simulink model "inverse_shapers"  (R2015b)
settings: Solver=ode1  StartTime=0.0  StopTime=30  FixedStep=0.001  RelTol=1e-3
undefined symbols (not defined in the file): a, A, tau, tau_add, tau_sub
libraries: cstblocks x1
settings Model: Creator=dave  LastModifiedBy=dave

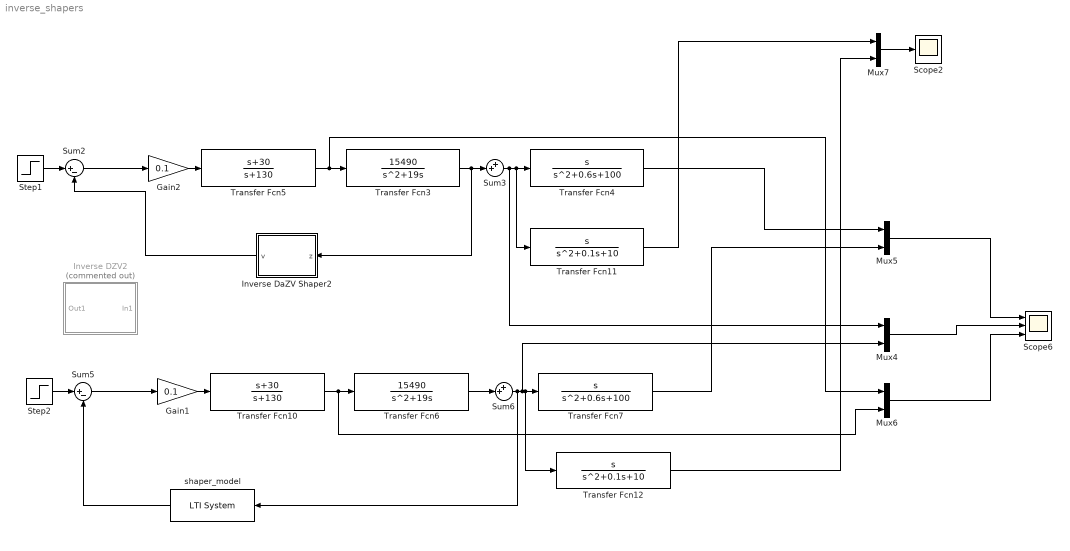
== system inverse_shapers ==
  Gain1 : Gain  Gain=0.1
  Gain2 : Gain  Gain=0.1
  Inverse DZV2 : Subsystem  Commented=on
  Inverse DaZV Shaper2 : Subsystem
  Mux{4..7} (4 alike) : Mux  Inputs=2
  Scope2 : Scope
  Scope6 : Scope  NumInputPorts=3
  Step1 : Step  SampleTime=0
  Step2 : Step  SampleTime=0
  Sum2 : Sum  Inputs=|+-
  Sum3 : Sum  Inputs=++|
  Sum5 : Sum  Inputs=|+-
  Sum6 : Sum  Inputs=++|
  Transfer Fcn10 : TransferFcn  Numerator=[1 30]  Denominator=[1 130]
  Transfer Fcn11 : TransferFcn  Numerator=[1 0]  Denominator=[1 0.1 10]
  Transfer Fcn12 : TransferFcn  Numerator=[1 0]  Denominator=[1 0.1 10]
  Transfer Fcn3 : TransferFcn  Numerator=[15490]  Denominator="[1  19 0]"
  Transfer Fcn4 : TransferFcn  Numerator=[1 0]  Denominator=[1 0.6 100]
  Transfer Fcn5 : TransferFcn  Numerator=[1 30]  Denominator=[1 130]
  Transfer Fcn6 : TransferFcn  Numerator=[15490]  Denominator="[1  19 0]"
  Transfer Fcn7 : TransferFcn  Numerator=[1 0]  Denominator=[1 0.6 100]
  shaper_model : cstblocks/LTI System  sys=ssi  IC=[]
  wires:
  Transfer Fcn5/1 -> Mux6/1, Transfer Fcn3/1
  Sum2/1 -> Gain2/1
  Step1/1 -> Sum2/1
  Transfer Fcn4/1 -> Mux5/1
  Gain2/1 -> Transfer Fcn5/1
  Transfer Fcn10/1 -> Mux6/2, Transfer Fcn6/1
  Transfer Fcn6/1 -> Sum6/2
  Sum5/1 -> Gain1/1
  Step2/1 -> Sum5/1
  Gain1/1 -> Transfer Fcn10/1
  Mux4/1 -> Scope6/2
  Mux5/1 -> Scope6/1
  Transfer Fcn7/1 -> Mux5/2
  Mux6/1 -> Scope6/3
  Transfer Fcn11/1 -> Mux7/1
  Mux7/1 -> Scope2/1
  Sum3/1 -> Mux4/1, Transfer Fcn11/1, Transfer Fcn4/1
  Transfer Fcn3/1 -> Inverse DaZV Shaper2/1(z), Sum3/2
  shaper_model/1 -> Sum5/2
  Transfer Fcn12/1 -> Mux7/2
  Inverse DaZV Shaper2/1(v) -> Sum2/2
  Sum6/1 -> shaper_model/1, Mux4/2, Transfer Fcn12/1, Transfer Fcn7/1

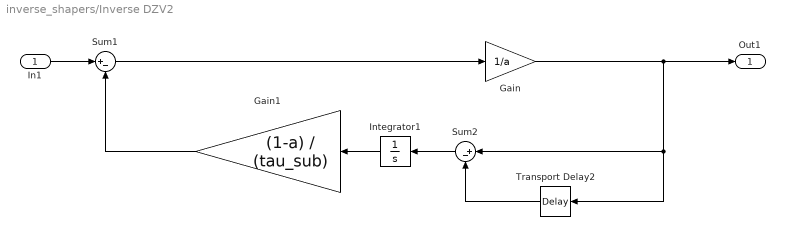
== system inverse_shapers/Inverse DZV2 ==
  In1 : Inport
  Gain : Gain  Gain=1/a
  Gain1 : Gain  Gain=(1-a) / (tau_sub)
  Integrator1 : Integrator  LimitOutput=on  UpperSaturationLimit=tau  LowerSaturationLimit=0
  Sum1 : Sum  Inputs=|+-
  Sum2 : Sum  Inputs=|+-
  Transport Delay2 : TransportDelay  DelayTime=tau_sub
  Out1 : Outport
  wires:
  Sum2/1 -> Integrator1/1
  Sum1/1 -> Gain/1
  In1/1 -> Sum1/1
  Transport Delay2/1 -> Sum2/2
  Gain/1 -> Sum2/1, Transport Delay2/1, Out1/1
  Integrator1/1 -> Gain1/1
  Gain1/1 -> Sum1/2

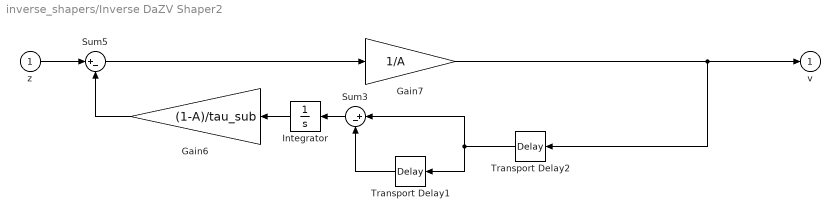
== system inverse_shapers/Inverse DaZV Shaper2 ==
  z : Inport
  Gain6 : Gain  Gain=(1-A)/tau_sub
  Gain7 : Gain  Gain=1/A
  Integrator : Integrator
  Sum3 : Sum  Inputs=|+-
  Sum5 : Sum  Inputs=|+-
  Transport Delay1 : TransportDelay  DelayTime=tau_sub
  Transport Delay2 : TransportDelay  DelayTime=tau_add
  v : Outport
  wires:
  z/1 -> Sum5/1
  Transport Delay1/1 -> Sum3/2
  Sum3/1 -> Integrator/1
  Integrator/1 -> Gain6/1
  Sum5/1 -> Gain7/1
  Gain7/1 -> Transport Delay2/1, v/1
  Gain6/1 -> Sum5/2
  Transport Delay2/1 -> Sum3/1, Transport Delay1/1
